simulink library "TestLibrary_LIB"  (R2018a)
settings: Solver=VariableStepAuto  StartTime=0.0  StopTime=10.0  RelTol=1e-3
settings Model: Creator=Choaib ELMADI  LastModifiedBy=Choaib ELMADI

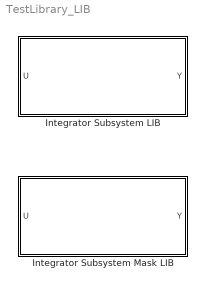
== system TestLibrary_LIB ==
  Integrator Subsystem LIB : Subsystem
  Integrator Subsystem Mask LIB : Subsystem  mask{FF=.03, FB=.97}
      mask prompts: FF "Feedforward Gain"; FB "Feedback Gain"

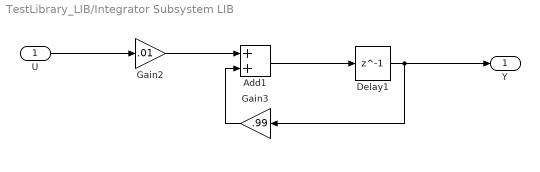
== system TestLibrary_LIB/Integrator Subsystem LIB ==
  U : Inport
  Add1 : Sum
  Delay1 : Delay  DelayLength=1
  Gain2 : Gain  Gain=.01
  Gain3 : Gain  Gain=.99
  Y : Outport
  wires:
  U/1 -> Gain2/1
  Add1/1 -> Delay1/1
  Gain2/1 -> Add1/1
  Delay1/1 -> Gain3/1, Y/1
  Gain3/1 -> Add1/2

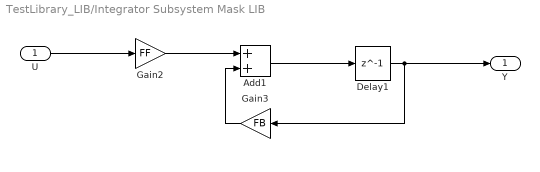
== system TestLibrary_LIB/Integrator Subsystem Mask LIB ==
  U : Inport
  Add1 : Sum
  Delay1 : Delay  DelayLength=1
  Gain2 : Gain  Gain=FF
  Gain3 : Gain  Gain=FB
  Y : Outport
  wires:
  Gain3/1 -> Add1/2
  Delay1/1 -> Y/1, Gain3/1
  Gain2/1 -> Add1/1
  Add1/1 -> Delay1/1
  U/1 -> Gain2/1
